simulink model "ProvNavModel"  (R2023b)
settings: Solver=ode5  StartTime=0.0  StopTime=tf  FixedStep=dt  RelTol=1e-3
values from neighbouring files (symbols this model uses):
  missDistanceThreshold = 1    [Main.m]
  mslPosX0 = 0    [Main.m]
  mslPosY0 = 0    [Main.m]
  mslVelX0 = 10    [Main.m]
  mslVelY0 = 0    [Main.m]
  proNavConst = 30    [Main.m]
  tgtPosX0 = 300.0    (= 300)    [Main.m]
  tgtPosY0 = 60.0    (= 60)    [Main.m]
  tgtVelX0 = 5    [Main.m]
  tgtVelY0 = 5    [Main.m]
settings Model: Creator=cmonti  LastModifiedBy=cmonti
settings DataIOCC: SaveFormat=Array  SaveOutput=off  SignalLogging=off  DSMLogging=off  ReturnWorkspaceOutputs=off

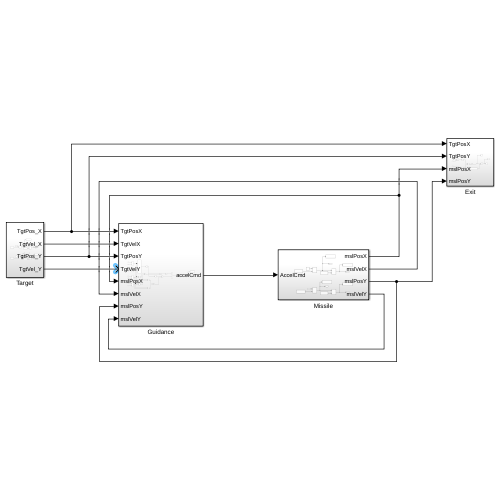
[thumbnail: Simulink's stored preview of the top-level diagram]
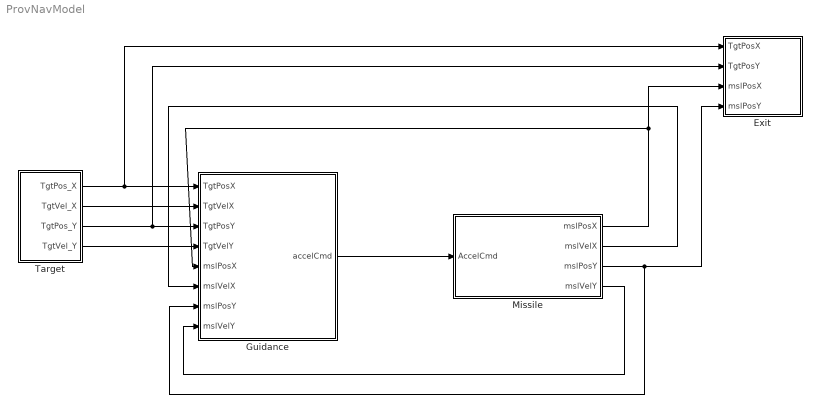
== system ProvNavModel ==
  Exit : Subsystem
  Guidance : Subsystem
  Missile : Subsystem
  Target : Subsystem
  wires:
  Guidance/1(accelCmd) -> Missile/1(AccelCmd)
  Missile/2(mslVelX) -> Guidance/6(mslVelX)
  Missile/3(mslPosY) -> Exit/4(mslPosY), Guidance/7(mslPosY)
  Target/1(TgtPos_X) -> Exit/1(TgtPosX), Guidance/1(TgtPosX)
  Target/3(TgtPos_Y) -> Exit/2(TgtPosY), Guidance/3(TgtPosY)
  Missile/1(mslPosX) -> Exit/3(mslPosX), Guidance/5(mslPosX)
  Missile/4(mslVelY) -> Guidance/8(mslVelY)
  Target/2(TgtVel_X) -> Guidance/2(TgtVelX)
  Target/4(TgtVel_Y) -> Guidance/4(TgtVelY)

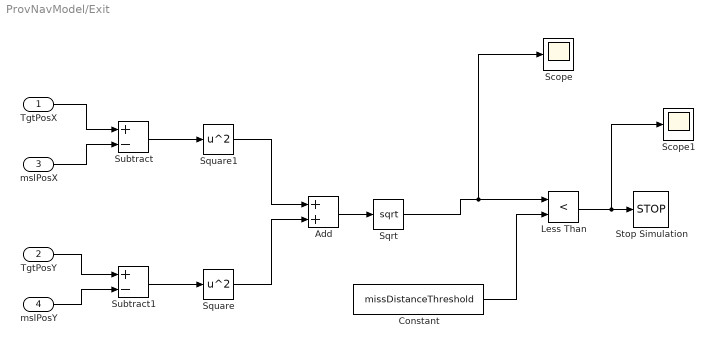
== system ProvNavModel/Exit ==
  TgtPosX : Inport
  TgtPosY : Inport  Port=2
  mslPosX : Inport  Port=3
  mslPosY : Inport  Port=4
  Add : Sum
  Constant : Constant  Value=missDistanceThreshold
  Less Than : RelationalOperator  Operator=<  OutDataTypeStr=boolean  RndMeth=Simplest  InputSameDT=off
  Scope : Scope
  Scope1 : Scope
  Sqrt : Sqrt
  Square : Math  Operator=square
  Square1 : Math  Operator=square
  Stop Simulation : Stop
  Subtract : Sum  Inputs=+-
  Subtract1 : Sum  Inputs=+-
  wires:
  TgtPosX/1 -> Subtract/1
  mslPosX/1 -> Subtract/2
  TgtPosY/1 -> Subtract1/1
  mslPosY/1 -> Subtract1/2
  Subtract1/1 -> Square/1
  Subtract/1 -> Square1/1
  Square1/1 -> Add/1
  Square/1 -> Add/2
  Constant/1 -> Less Than/2
  Add/1 -> Sqrt/1
  Sqrt/1 -> Scope/1, Less Than/1
  Less Than/1 -> Scope1/1, Stop Simulation/1

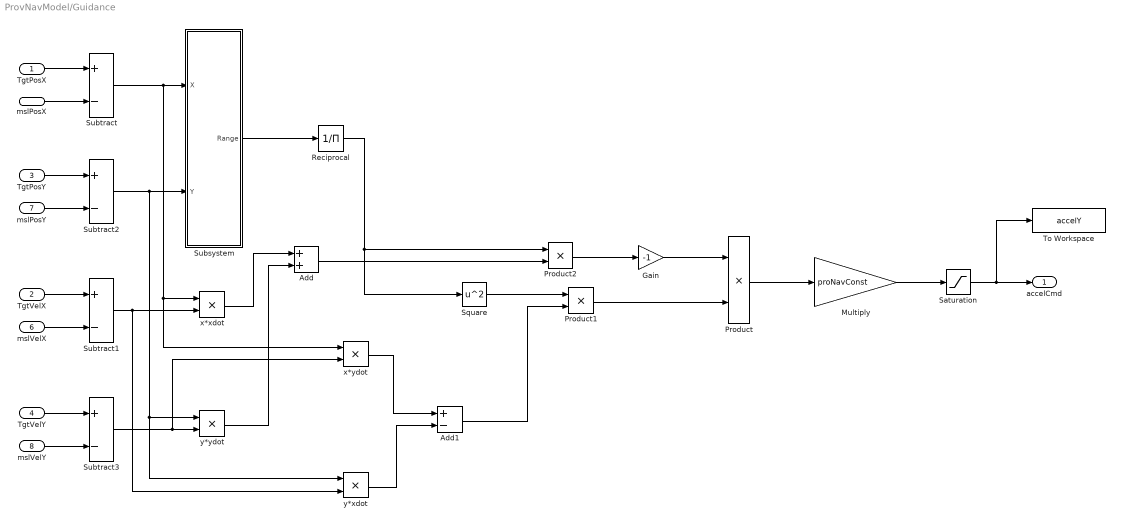
== system ProvNavModel/Guidance ==
  TgtPosX : Inport
  TgtVelX : Inport  Port=2
  TgtPosY : Inport  Port=3
  TgtVelY : Inport  Port=4
  mslPosX : Inport  Port=5
  mslVelX : Inport  Port=6
  mslPosY : Inport  Port=7
  mslVelY : Inport  Port=8
  Add : Sum
  Add1 : Sum  Inputs=+-
  Gain : Gain  Gain=-1
  Multiply : Gain  Gain=proNavConst
  Product : Product
  Product1 : Product
  Product2 : Product
  Reciprocal : Product  Inputs=/
  Saturation : Saturate  UpperLimit=50  LowerLimit=-50
  Square : Math  Operator=square
  Subsystem : Subsystem
  Subtract{,1..3} (4 alike) : Sum  Inputs=+-
  To Workspace : ToWorkspace  VariableName=accelY  SampleTime=-1
  x*xdot : Product
  x*ydot : Product
  y*xdot : Product
  y*ydot : Product
  accelCmd : Outport
  wires:
  Multiply/1 -> Saturation/1
  Product/1 -> Multiply/1
  TgtVelX/1 -> Subtract1/1
  mslVelX/1 -> Subtract1/2
  TgtVelY/1 -> Subtract3/1
  mslVelY/1 -> Subtract3/2
  Gain/1 -> Product/1
  Subtract/1 -> Subsystem/1(X), x*ydot/1, x*xdot/1
  Subtract2/1 -> Subsystem/2(Y), y*xdot/1, y*ydot/1
  mslPosY/1 -> Subtract2/2
  TgtPosY/1 -> Subtract2/1
  mslPosX/1 -> Subtract/2
  TgtPosX/1 -> Subtract/1
  Subsystem/1(Range) -> Reciprocal/1
  Square/1 -> Product1/1
  Reciprocal/1 -> Product2/1, Square/1
  Product1/1 -> Product/2
  Product2/1 -> Gain/1
  x*xdot/1 -> Add/1
  y*ydot/1 -> Add/2
  Add/1 -> Product2/2
  Add1/1 -> Product1/2
  Subtract1/1 -> x*xdot/2, y*xdot/2
  Subtract3/1 -> x*ydot/2, y*ydot/2
  x*ydot/1 -> Add1/1
  y*xdot/1 -> Add1/2
  Saturation/1 -> To Workspace/1, accelCmd/1

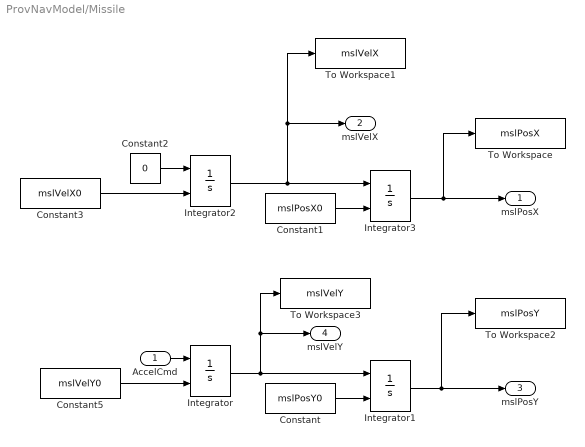
== system ProvNavModel/Missile ==
  AccelCmd : Inport
  Constant : Constant  Value=mslPosY0
  Constant1 : Constant  Value=mslPosX0
  Constant2 : Constant  Value=0
  Constant3 : Constant  Value=mslVelX0
  Constant5 : Constant  Value=mslVelY0
  Integrator{,1..3} (4 alike) : Integrator  InitialConditionSource=external
  To Workspace : ToWorkspace  VariableName=mslPosX  SampleTime=-1
  To Workspace1 : ToWorkspace  VariableName=mslVelX  SampleTime=-1
  To Workspace2 : ToWorkspace  VariableName=mslPosY  SampleTime=-1
  To Workspace3 : ToWorkspace  VariableName=mslVelY  SampleTime=-1
  mslPosX : Outport
  mslVelX : Outport  Port=2
  mslPosY : Outport  Port=3
  mslVelY : Outport  Port=4
  wires:
  Integrator1/1 -> To Workspace2/1, mslPosY/1
  AccelCmd/1 -> Integrator/1
  Integrator/1 -> mslVelY/1, To Workspace3/1, Integrator1/1
  Constant/1 -> Integrator1/2
  Constant1/1 -> Integrator3/2
  Constant2/1 -> Integrator2/1
  Constant3/1 -> Integrator2/2
  Constant5/1 -> Integrator/2
  Integrator3/1 -> mslPosX/1, To Workspace/1
  Integrator2/1 -> To Workspace1/1, mslVelX/1, Integrator3/1

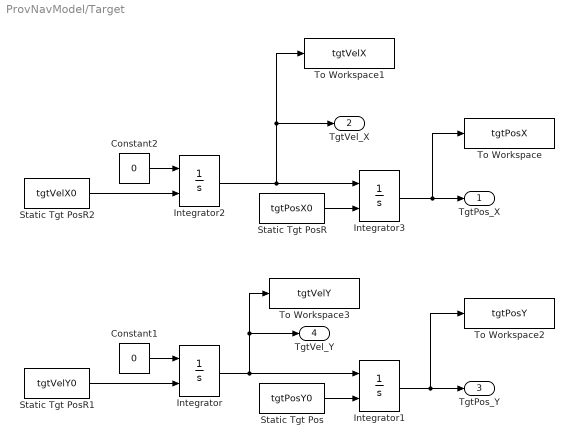
== system ProvNavModel/Target ==
  Constant1 : Constant  Value=0
  Constant2 : Constant  Value=0
  Integrator{,1..3} (4 alike) : Integrator  InitialConditionSource=external
  Static Tgt Pos : Constant  Value=tgtPosY0
  Static Tgt PosR : Constant  Value=tgtPosX0
  Static Tgt PosR1 : Constant  Value=tgtVelY0
  Static Tgt PosR2 : Constant  Value=tgtVelX0
  To Workspace : ToWorkspace  VariableName=tgtPosX  SampleTime=-1
  To Workspace1 : ToWorkspace  VariableName=tgtVelX  SampleTime=-1
  To Workspace2 : ToWorkspace  VariableName=tgtPosY  SampleTime=-1
  To Workspace3 : ToWorkspace  VariableName=tgtVelY  SampleTime=-1
  TgtPos_X : Outport
  TgtVel_X : Outport  Port=2
  TgtPos_Y : Outport  Port=3
  TgtVel_Y : Outport  Port=4
  wires:
  Static Tgt PosR/1 -> Integrator3/2
  Integrator2/1 -> TgtVel_X/1, To Workspace1/1, Integrator3/1
  Constant2/1 -> Integrator2/1
  Static Tgt Pos/1 -> Integrator1/2
  Integrator/1 -> TgtVel_Y/1, To Workspace3/1, Integrator1/1
  Integrator1/1 -> TgtPos_Y/1, To Workspace2/1
  Static Tgt PosR1/1 -> Integrator/2
  Static Tgt PosR2/1 -> Integrator2/2
  Integrator3/1 -> TgtPos_X/1, To Workspace/1
  Constant1/1 -> Integrator/1

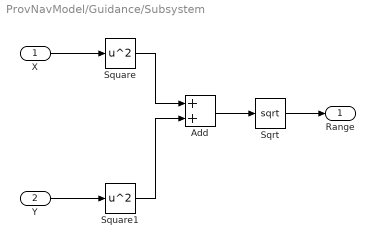
== system ProvNavModel/Guidance/Subsystem ==
  X : Inport
  Y : Inport  Port=2
  Add : Sum
  Sqrt : Sqrt
  Square : Math  Operator=square
  Square1 : Math  Operator=square
  Range : Outport
  wires:
  Square/1 -> Add/1
  Square1/1 -> Add/2
  Sqrt/1 -> Range/1
  Add/1 -> Sqrt/1
  X/1 -> Square/1
  Y/1 -> Square1/1
